simulink model "main_adaptive"  (R2021b)
settings: Solver=ode45  StartTime=0.0  StopTime=80  FixedStep=0.1  RelTol=1e-4
libraries: slpidlib x6
(part 1 of 2)
settings Model: Creator=rooz1200  LastModifiedBy=rooz1200
settings SolverCC: AlgebraicLoopSolver=TrustRegion
settings OptimizationCC: DefaultParameterBehavior=Inlined  EnhancedBackFolding=on  PassReuseOutputArgsAs=Individual arguments  ZeroExternalMemoryAtStartup=off  ZeroInternalMemoryAtStartup=off  OptimizeBlockOrder=speed  DifferentSizesBufferReuse=on  OptimizationCustomize=off  EfficientTunableParamExpr=on
settings DebuggingCC: ParameterTunabilityLossMsg=error  UnderSpecifiedDimensionMsg=warning  ArithmeticOperatorsInVariantConditions=warning
settings SFSimCC: MATLABDynamicMemAlloc=off  CustomCodeUndefinedFunction=UseInterfaceOnly
settings RTWCC: Description=Embedded Coder  SystemTargetFile=ert.tlc  GenCodeOnly=on  TemplateMakefile=ert_default_tmf
settings CodeAppCC: ForceParamTrailComments=on  IgnoreCustomStorageClasses=off  OperatorAnnotations=on  SimulinkDataObjDesc=on  SFDataObjDesc=on  InsertBlockDesc=on
settings ERTTargetCC: TargetLangStandard=C99 (ISO)  GenerateSampleERTMain=on  InlinedParameterPlacement=NonHierarchical  ERTCustomFileTemplate=example_file_process.tlc

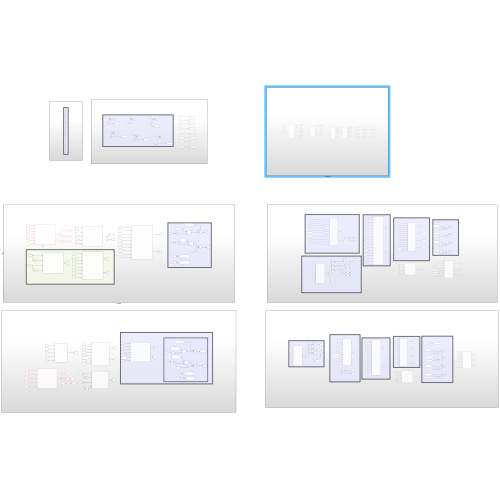
[thumbnail: Simulink's stored preview of the top-level diagram]
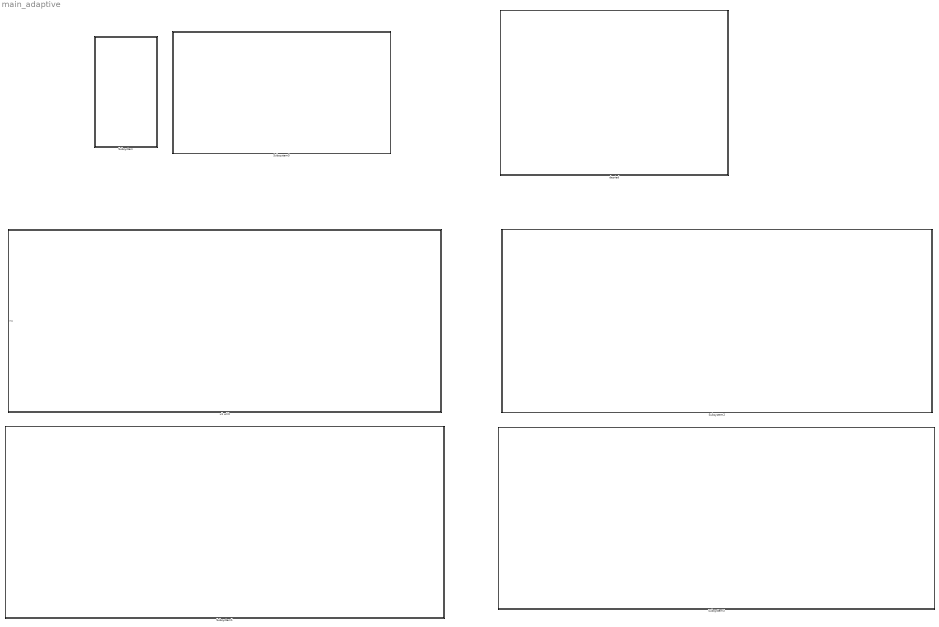
== system main_adaptive ==
  Subsystem : Subsystem
  Subsystem1 : Subsystem
  Subsystem2 : Subsystem
  Subsystem3 : Subsystem
  Subsystem5 : Subsystem
  desried : Subsystem
  "u1 whit " : Subsystem

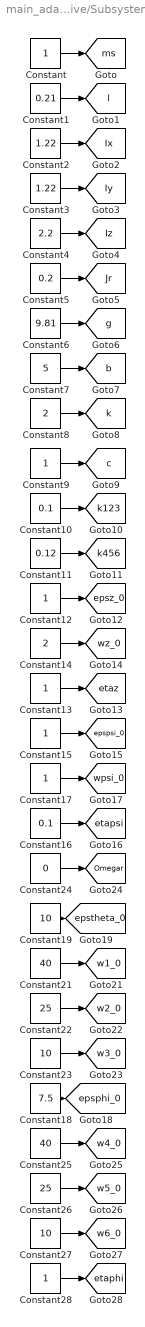
== system main_adaptive/Subsystem ==
  Constant{,9,12..13,15,17,28} (7 alike) : Constant
  Constant1 : Constant  Value=0.21
  Constant10 : Constant  Value=0.1
  Constant11 : Constant  Value=0.12
  Constant14 : Constant  Value=2
  Constant16 : Constant  Value=0.1
  Constant18 : Constant  Value=7.5
  Constant19 : Constant  Value=10
  Constant2 : Constant  Value=1.22
  Constant21 : Constant  Value=40
  Constant22 : Constant  Value=25
  Constant23 : Constant  Value=10
  Constant24 : Constant  Value=0
  Constant25 : Constant  Value=40
  Constant26 : Constant  Value=25
  Constant27 : Constant  Value=10
  Constant3 : Constant  Value=1.22
  Constant4 : Constant  Value=2.2
  Constant5 : Constant  Value=0.2
  Constant6 : Constant  Value=9.81
  Constant7 : Constant  Value=5
  Constant8 : Constant  Value=2
  tag scope: Ix=global, Iy=global, Iz=global, Jr=global, Omegar=global, b=global, c=global, epsphi_0=global, epspsi_0=global, epstheta_0=global, epsz_0=global, etaphi=global, etapsi=global, etaz=global, g=global, k123=global, k456=global, k=global, l=global, ms=global, w1_0=global, w2_0=global, w3_0=global, w4_0=global, w5_0=global, w6_0=global, wpsi_0=global, wz_0=global
  wires:
  Constant15/1 -> [epspsi_0]
  Constant4/1 -> [Iz]
  Constant11/1 -> [k456]
  Constant/1 -> [ms]
  Constant10/1 -> [k123]
  Constant22/1 -> [w2_0]
  Constant1/1 -> [l]
  Constant6/1 -> [g]
  Constant17/1 -> [wpsi_0]
  Constant13/1 -> [etaz]
  Constant21/1 -> [w1_0]
  Constant8/1 -> [k]
  Constant25/1 -> [w4_0]
  Constant23/1 -> [w3_0]
  Constant18/1 -> [epsphi_0]
  Constant3/1 -> [Iy]
  Constant2/1 -> [Ix]
  Constant16/1 -> [etapsi]
  Constant24/1 -> [Omegar]
  Constant26/1 -> [w5_0]
  Constant5/1 -> [Jr]
  Constant7/1 -> [b]
  Constant19/1 -> [epstheta_0]
  Constant14/1 -> [wz_0]
  Constant27/1 -> [w6_0]
  Constant12/1 -> [epsz_0]
  Constant9/1 -> [c]
  Constant28/1 -> [etaphi]

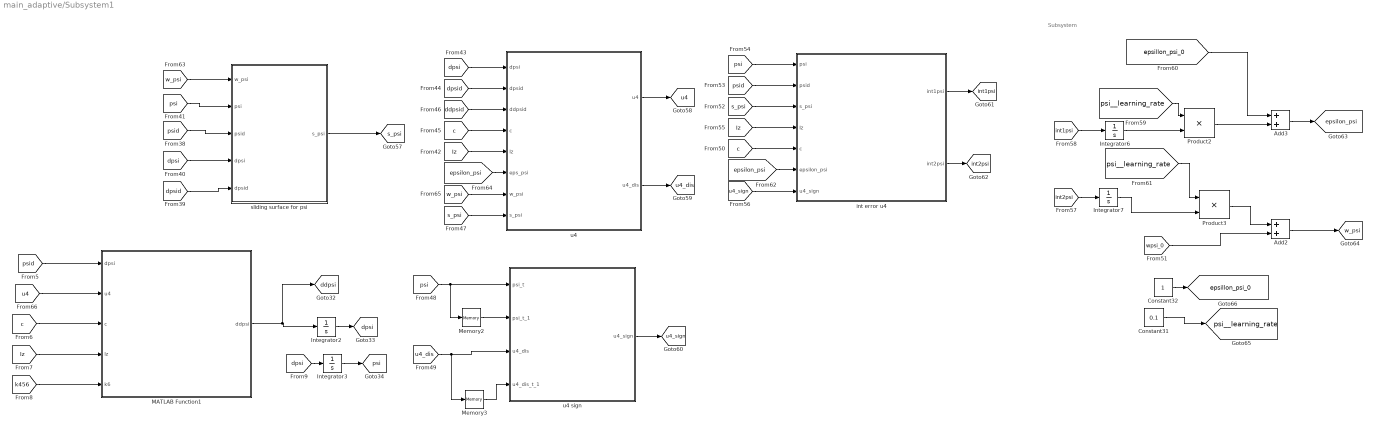
== system main_adaptive/Subsystem1 ==
  note: Subsystem
  Add2 : Sum
  Add3 : Sum
  Constant31 : Constant  Value=0.1
  Constant32 : Constant
  Integrator{2..3,6..7} (4 alike) : Integrator
  MATLAB Function1 : MATLAB Function  TreatAsAtomicUnit=on
  Memory2 : Memory
  Memory3 : Memory
  Product2 : Product
  Product3 : Product
  int error u4 : MATLAB Function  TreatAsAtomicUnit=on
  sliding surface for psi : MATLAB Function  TreatAsAtomicUnit=on
  u4 : MATLAB Function  TreatAsAtomicUnit=on
  "u4 sign " : MATLAB Function  TreatAsAtomicUnit=on
  tag scope: ddpsi=global, dpsi=global, epsillon_psi_0=global, epsilon_psi=global, int1psi=global, int2psi=global, psi=global, psi__learning_rate=global, s_psi=global, u4=global, u4_dis=global, u4_sign=global, w_psi=global
  wires:
  [psid] -> int error u4/2(psid)
  [dpsi] -> u4/1(dpsi)
  [c] -> int error u4/5(c)
  [u4_dis] -> "u4 sign "/3(u4_dis), Memory3/1
  "u4 sign "/1(u4_sign) -> [u4_sign]
  [psi] -> sliding surface for psi/2(psi)
  [w_psi] -> u4/7(w_psi)
  [dpsid] -> sliding surface for psi/5(dpsid)
  [u4_sign] -> int error u4/7(u4_sign)
  [epsilon_psi] -> int error u4/6(epsilon_psi)
  [epsilon_psi] -> u4/6(eps_psi)
  Memory3/1 -> "u4 sign "/4(u4_dis_t_1)
  sliding surface for psi/1(s_psi) -> [s_psi]
  [c] -> u4/4(c)
  [dpsi] -> sliding surface for psi/4(dpsi)
  [s_psi] -> u4/8(s_psi)
  [psi] -> int error u4/1(psi)
  u4/1(u4) -> [u4]
  [s_psi] -> int error u4/3(s_psi)
  Memory2/1 -> "u4 sign "/2(psi_t_1)
  [psi] -> "u4 sign "/1(psi_t), Memory2/1
  int error u4/1(int1psi) -> [int1psi]
  int error u4/2(int2psi) -> [int2psi]
  [ddpsid] -> u4/3(ddpsid)
  [Iz] -> int error u4/4(Iz)
  [w_psi] -> sliding surface for psi/1(w_psi)
  u4/2(u4_dis) -> [u4_dis]
  [psid] -> sliding surface for psi/3(psid)
  [dpsid] -> u4/2(dpsid)
  [Iz] -> u4/5(Iz)
  Constant32/1 -> [epsillon_psi_0]
  [psi__learning_rate] -> Product2/1
  Integrator6/1 -> Product2/2
  Product3/1 -> Add2/1
  [int1psi] -> Integrator6/1
  Add2/1 -> [w_psi]
  [wpsi_0] -> Add2/2
  Add3/1 -> [epsilon_psi]
  Integrator7/1 -> Product3/2
  [psi__learning_rate] -> Product3/1
  [int2psi] -> Integrator7/1
  Constant31/1 -> [psi__learning_rate]
  Product2/1 -> Add3/2
  [epsillon_psi_0] -> Add3/1
  [k456] -> MATLAB Function1/5(k6)
  [Iz] -> MATLAB Function1/4(Iz)
  [c] -> MATLAB Function1/3(c)
  Integrator3/1 -> [psi]
  [psid] -> MATLAB Function1/1(dpsi)
  [u4] -> MATLAB Function1/2(u4)
  MATLAB Function1/1(ddpsi) -> [ddpsi], Integrator2/1
  Integrator2/1 -> [dpsi]
  [dpsi] -> Integrator3/1

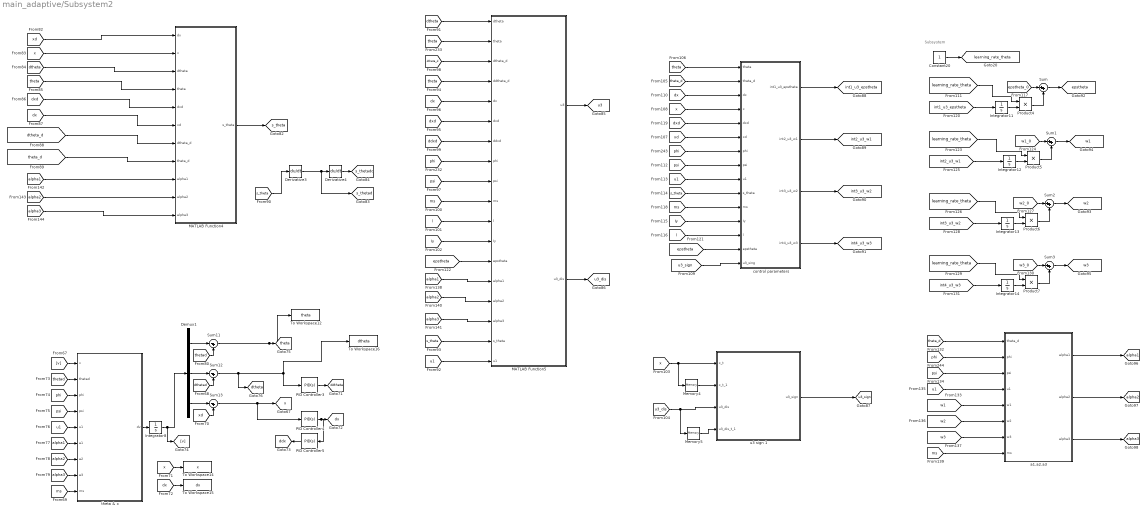
== system main_adaptive/Subsystem2 ==
  note: Subsystem
  Constant20 : Constant
  Demux1 : Demux  Outputs=3
  Derivative3 : Derivative
  Derivative4 : Derivative
  Integrator{11..14} (4 alike) : Integrator
  Integrator8 : Integrator  InitialCondition=[0;0;0.6]
  MATLAB Function4 : MATLAB Function  TreatAsAtomicUnit=on
  MATLAB Function5 : MATLAB Function  TreatAsAtomicUnit=on
  Memory4 : Memory
  Memory5 : Memory
  PID Controller3 : slpidlib/PID Controller  Controller=PID  Form=Parallel  TimeDomain=Continuous-time  UseExternalTs=off  SampleTime=-1  IntegratorMethod=Forward Euler  FilterMethod=Forward Euler  ControllerParametersSource=internal  P=0  I=0  D=1  UseFilter=on  N=100  TunerSelectOption=Transfer Function Based (PID Tuner App)  InitialConditionSource=internal  InitialConditionForIntegrator=0  InitialConditionForFilter=0  DifferentiatorICPrevScaledInput=0  ExternalReset=none  TrackingMode=off  Kt=1  LimitOutput=off  SatLimitsSource=internal  UpperSaturationLimit=inf  LowerSaturationLimit=-inf  LinearizeAsGain=on  AntiWindupMode=none  Kb=1  POutMin=[]  POutMax=[]  IOutMin=[]  IOutMax=[]  DOutMin=[]  DOutMax=[]  NOutMin=[]  NOutMax=[]  SumOutMin=[]  SumOutMax=[]  SaturationOutMin=[]  SaturationOutMax=[]  PParamMin=[]  PParamMax=[]  IParamMin=[]  IParamMax=[]  DParamMin=[]  DParamMax=[]  NParamMin=[]  NParamMax=[]  KbParamMin=[]  KbParamMax=[]  KtParamMin=[]  KtParamMax=[]  KbOutMin=[]  KbOutMax=[]  KtOutMin=[]  KtOutMax=[]  IntegratorOutMin=[]  IntegratorOutMax=[]  FilterOutMin=[]  FilterOutMax=[]  SumI1OutMin=[]  SumI1OutMax=[]  SumI2OutMin=[]  SumI2OutMax=[]  SumI3OutMin=[]  SumI3OutMax=[]  SumI4OutMin=[]  SumI4OutMax=[]  SumDOutMin=[]  SumDOutMax=[]  DifferentiatorOutMin=[]  DifferentiatorOutMax=[]  FilterDiffOutCoefMin=[]  FilterDiffOutCoefMax=[]  ReciprocalOutMin=[]  ReciprocalOutMax=[]  SumDenOutMin=[]  SumDenOutMax=[]  SumNumOutMin=[]  SumNumOutMax=[]  DivideOutMin=[]  DivideOutMax=[]  UdiffTsProdOutMin=[]  UdiffTsProdOutMax=[]  NTsProdOutMin=[]  NTsProdOutMax=[]  UintegralTsProdOutMin=[]  UintegralTsProdOutMax=[]  UngainTsProdOutMin=[]  UngainTsProdOutMax=[]  IntegratorContinuousStateAttributes=''  IntegratorStateMustResolveToSignalObject=off  IntegratorRTWStateStorageClass=Auto  FilterContinuousStateAttributes=''  FilterStateMustResolveToSignalObject=off  FilterRTWStateStorageClass=Auto  ParallelPVariant=InternalParameters  IdealPVariant=Disabled  IVariant=InternalParameters  DVariant=InternalParameters  IntegratorVariant=Continuous  SatVariant=Disabled  AWVariant=Passthrough  PCopyVariant=Disabled  TRVariant=Disabled  FdbkBlocksVariant=Forward  IdealPFdbkVariant=Disabled  SatFdbkVariant=Disabled  DerivativeFilterVariant=ContFilter  NVariant=InternalParameters  NCopyVariant=Disabled  FilterICVariant=InternalICsFilter  IntegratorICVariant=InternalICs  ExternalResetVariant=Disabled  TRSumVariant=Passthrough  SumFdbkVariant=Disabled  SumVariant=Sum_PID  TsampFilterVariant=InternalTs  TsampNgainVariant=Passthrough  TsampIntegralVariant=Passthrough  ExternalSaturationOutDataTypeStr=Inherit: Same as second input
  PID Controller4 : slpidlib/PID Controller  Controller=PID  Form=Parallel  TimeDomain=Continuous-time  UseExternalTs=off  SampleTime=-1  IntegratorMethod=Forward Euler  FilterMethod=Forward Euler  ControllerParametersSource=internal  P=0  I=0  D=1  UseFilter=on  N=100  TunerSelectOption=Transfer Function Based (PID Tuner App)  InitialConditionSource=internal  InitialConditionForIntegrator=0  InitialConditionForFilter=0  DifferentiatorICPrevScaledInput=0  ExternalReset=none  TrackingMode=off  Kt=1  LimitOutput=off  SatLimitsSource=internal  UpperSaturationLimit=inf  LowerSaturationLimit=-inf  LinearizeAsGain=on  AntiWindupMode=none  Kb=1  POutMin=[]  POutMax=[]  IOutMin=[]  IOutMax=[]  DOutMin=[]  DOutMax=[]  NOutMin=[]  NOutMax=[]  SumOutMin=[]  SumOutMax=[]  SaturationOutMin=[]  SaturationOutMax=[]  PParamMin=[]  PParamMax=[]  IParamMin=[]  IParamMax=[]  DParamMin=[]  DParamMax=[]  NParamMin=[]  NParamMax=[]  KbParamMin=[]  KbParamMax=[]  KtParamMin=[]  KtParamMax=[]  KbOutMin=[]  KbOutMax=[]  KtOutMin=[]  KtOutMax=[]  IntegratorOutMin=[]  IntegratorOutMax=[]  FilterOutMin=[]  FilterOutMax=[]  SumI1OutMin=[]  SumI1OutMax=[]  SumI2OutMin=[]  SumI2OutMax=[]  SumI3OutMin=[]  SumI3OutMax=[]  SumI4OutMin=[]  SumI4OutMax=[]  SumDOutMin=[]  SumDOutMax=[]  DifferentiatorOutMin=[]  DifferentiatorOutMax=[]  FilterDiffOutCoefMin=[]  FilterDiffOutCoefMax=[]  ReciprocalOutMin=[]  ReciprocalOutMax=[]  SumDenOutMin=[]  SumDenOutMax=[]  SumNumOutMin=[]  SumNumOutMax=[]  DivideOutMin=[]  DivideOutMax=[]  UdiffTsProdOutMin=[]  UdiffTsProdOutMax=[]  NTsProdOutMin=[]  NTsProdOutMax=[]  UintegralTsProdOutMin=[]  UintegralTsProdOutMax=[]  UngainTsProdOutMin=[]  UngainTsProdOutMax=[]  IntegratorContinuousStateAttributes=''  IntegratorStateMustResolveToSignalObject=off  IntegratorRTWStateStorageClass=Auto  FilterContinuousStateAttributes=''  FilterStateMustResolveToSignalObject=off  FilterRTWStateStorageClass=Auto  ParallelPVariant=InternalParameters  IdealPVariant=Disabled  IVariant=InternalParameters  DVariant=InternalParameters  IntegratorVariant=Continuous  SatVariant=Disabled  AWVariant=Passthrough  PCopyVariant=Disabled  TRVariant=Disabled  FdbkBlocksVariant=Forward  IdealPFdbkVariant=Disabled  SatFdbkVariant=Disabled  DerivativeFilterVariant=ContFilter  NVariant=InternalParameters  NCopyVariant=Disabled  FilterICVariant=InternalICsFilter  IntegratorICVariant=InternalICs  ExternalResetVariant=Disabled  TRSumVariant=Passthrough  SumFdbkVariant=Disabled  SumVariant=Sum_PID  TsampFilterVariant=InternalTs  TsampNgainVariant=Passthrough  TsampIntegralVariant=Passthrough  ExternalSaturationOutDataTypeStr=Inherit: Same as second input
  PID Controller5 : slpidlib/PID Controller  Controller=PID  Form=Parallel  TimeDomain=Continuous-time  UseExternalTs=off  SampleTime=-1  IntegratorMethod=Forward Euler  FilterMethod=Forward Euler  ControllerParametersSource=internal  P=0  I=0  D=1  UseFilter=on  N=100  TunerSelectOption=Transfer Function Based (PID Tuner App)  InitialConditionSource=internal  InitialConditionForIntegrator=0  InitialConditionForFilter=0  DifferentiatorICPrevScaledInput=0  ExternalReset=none  TrackingMode=off  Kt=1  LimitOutput=off  SatLimitsSource=internal  UpperSaturationLimit=inf  LowerSaturationLimit=-inf  LinearizeAsGain=on  AntiWindupMode=none  Kb=1  POutMin=[]  POutMax=[]  IOutMin=[]  IOutMax=[]  DOutMin=[]  DOutMax=[]  NOutMin=[]  NOutMax=[]  SumOutMin=[]  SumOutMax=[]  SaturationOutMin=[]  SaturationOutMax=[]  PParamMin=[]  PParamMax=[]  IParamMin=[]  IParamMax=[]  DParamMin=[]  DParamMax=[]  NParamMin=[]  NParamMax=[]  KbParamMin=[]  KbParamMax=[]  KtParamMin=[]  KtParamMax=[]  KbOutMin=[]  KbOutMax=[]  KtOutMin=[]  KtOutMax=[]  IntegratorOutMin=[]  IntegratorOutMax=[]  FilterOutMin=[]  FilterOutMax=[]  SumI1OutMin=[]  SumI1OutMax=[]  SumI2OutMin=[]  SumI2OutMax=[]  SumI3OutMin=[]  SumI3OutMax=[]  SumI4OutMin=[]  SumI4OutMax=[]  SumDOutMin=[]  SumDOutMax=[]  DifferentiatorOutMin=[]  DifferentiatorOutMax=[]  FilterDiffOutCoefMin=[]  FilterDiffOutCoefMax=[]  ReciprocalOutMin=[]  ReciprocalOutMax=[]  SumDenOutMin=[]  SumDenOutMax=[]  SumNumOutMin=[]  SumNumOutMax=[]  DivideOutMin=[]  DivideOutMax=[]  UdiffTsProdOutMin=[]  UdiffTsProdOutMax=[]  NTsProdOutMin=[]  NTsProdOutMax=[]  UintegralTsProdOutMin=[]  UintegralTsProdOutMax=[]  UngainTsProdOutMin=[]  UngainTsProdOutMax=[]  IntegratorContinuousStateAttributes=''  IntegratorStateMustResolveToSignalObject=off  IntegratorRTWStateStorageClass=Auto  FilterContinuousStateAttributes=''  FilterStateMustResolveToSignalObject=off  FilterRTWStateStorageClass=Auto  ParallelPVariant=InternalParameters  IdealPVariant=Disabled  IVariant=InternalParameters  DVariant=InternalParameters  IntegratorVariant=Continuous  SatVariant=Disabled  AWVariant=Passthrough  PCopyVariant=Disabled  TRVariant=Disabled  FdbkBlocksVariant=Forward  IdealPFdbkVariant=Disabled  SatFdbkVariant=Disabled  DerivativeFilterVariant=ContFilter  NVariant=InternalParameters  NCopyVariant=Disabled  FilterICVariant=InternalICsFilter  IntegratorICVariant=InternalICs  ExternalResetVariant=Disabled  TRSumVariant=Passthrough  SumFdbkVariant=Disabled  SumVariant=Sum_PID  TsampFilterVariant=InternalTs  TsampNgainVariant=Passthrough  TsampIntegralVariant=Passthrough  ExternalSaturationOutDataTypeStr=Inherit: Same as second input
  Product{4..7} (4 alike) : Product
  Sum{,1..3} (4 alike) : Sum  Inputs=|++
  Sum11 : Sum  Inputs=|-+
  Sum12 : Sum  Inputs=|-+
  Sum13 : Sum  Inputs=|-+
  To Workspace12 : ToWorkspace  VariableName=theta  SampleTime=-1
      settings: Save2DSignal=2-D array (concatenate along first dimension)
  To Workspace14 : ToWorkspace  VariableName=x  SampleTime=-1
      settings: Save2DSignal=2-D array (concatenate along first dimension)
  To Workspace15 : ToWorkspace  VariableName=dx  SampleTime=-1
      settings: Save2DSignal=2-D array (concatenate along first dimension)
  To Workspace16 : ToWorkspace  VariableName=dtheta  SampleTime=-1
      settings: Save2DSignal=2-D array (concatenate along first dimension)
  a1,a2,a3 : MATLAB Function  TreatAsAtomicUnit=on
  control parameters : MATLAB Function  TreatAsAtomicUnit=on
  theta & x : MATLAB Function  TreatAsAtomicUnit=on
  u3 sign 1 : MATLAB Function  TreatAsAtomicUnit=on
  tag scope: alpha1=global, alpha2=global, alpha3=global, ddtheta=global, ddx=global, dtheta=global, dx=global, epstheta=global, int1_u3_epstheta=global, int2_u3_w1=global, int3_u3_w2=global, int4_u3_w3=global, learning_rate_theta=global, s_theta=global, s_thetad=global, s_thetadd=global, theta=global, u3=global, u3_dis=global, u3_sign=global, w1=global, w2=global, w3=global, x=global
  wires:
  [dxd] -> MATLAB Function4/5(dxd)
  [alpha1] -> MATLAB Function4/9(alpha1)
  Memory4/1 -> u3 sign 1/2(x_t_1)
  [s_theta] -> MATLAB Function5/17(s_theta)
  Sum12/1 -> To Workspace16/1, PID Controller3/1, [dtheta]
  [theta] -> MATLAB Function5/2(theta)
  [phi] -> a1,a2,a3/2(phi)
  control parameters/4(int4_u3_w3) -> [int4_u3_w3]
  PID Controller5/1 -> [ddx]
  MATLAB Function5/1(u3) -> [u3]
  [ms] -> control parameters/11(ms)
  [theta] -> MATLAB Function5/4(ddtheta_d)
  [w2] -> a1,a2,a3/6(w2)
  Derivative4/1 -> [s_thetadd]
  [epstheta] -> control parameters/14(epstheta)
  [u3_sign] -> control parameters/15(u3_sing)
  [theta_d] -> control parameters/2(theta_d)
  [ms] -> MATLAB Function5/10(ms)
  [ddxd] -> MATLAB Function5/7(ddxd)
  Demux1/2 -> Sum12/1
  Sum11/1 -> To Workspace12/1, [theta]
  [theta_d] -> a1,a2,a3/1(theta_d)
  [alpha2] -> MATLAB Function4/10(alpha2)
  [thetad] -> Sum11/2
  [dxd] -> MATLAB Function5/6(dxd)
  [thetad] -> theta & x/2(thetad)
  a1,a2,a3/2(alpha2) -> [alpha2]
  [alpha1] -> MATLAB Function5/14(alpha1)
  [psi] -> theta & x/4(psi)
  [dtheta] -> MATLAB Function4/3(dtheta)
  Memory5/1 -> u3 sign 1/4(u3_dis_t_1)
  [ms] -> theta & x/9(ms)
  theta & x/1(dv) -> Integrator8/1
  [xd] -> control parameters/6(xd)
  Sum13/1 -> [x], PID Controller4/1
  [s_theta] -> Derivative3/1
  [alpha1] -> theta & x/6(a1)
  [phi] -> theta & x/3(phi)
  [dx] -> MATLAB Function5/5(dx)
  [psi] -> MATLAB Function5/9(psi)
  control parameters/3(int3_u3_w2) -> [int3_u3_w2]
  [alpha3] -> MATLAB Function4/11(alpha3)
  [x] -> u3 sign 1/1(x_t), Memory4/1
  [alpha2] -> MATLAB Function5/15(alpha2)
  [Iy] -> MATLAB Function5/12(Iy)
  [l] -> control parameters/13(l)
  [psi] -> control parameters/8(psi)
  [dtheta] -> MATLAB Function5/1(dtheta)
  MATLAB Function5/2(u3_dis) -> [u3_dis]
  MATLAB Function4/1(s_theta) -> [s_theta]
  [dtheta_d] -> MATLAB Function4/7(dtheta_d)
  [Iy] -> control parameters/12(Iy)
  [x] -> control parameters/4(x)
  [u1] -> control parameters/9(u1)
  [dtheta_d] -> MATLAB Function5/3(dtheta_d)
  [u1] -> MATLAB Function5/18(u1)
  [dx] -> MATLAB Function4/6(xd)
  control parameters/1(int1_u3_epstheta) -> [int1_u3_epstheta]
  [theta] -> MATLAB Function4/4(theta)
  [phi] -> MATLAB Function5/8(phi)
  [dthetad] -> Sum12/2
  [ms] -> a1,a2,a3/8(ms)
  control parameters/2(int2_u3_w1) -> [int2_u3_w1]
  [u3_dis] -> u3 sign 1/3(u3_dis), Memory5/1
  Derivative3/1 -> Derivative4/1, [s_thetad]
  a1,a2,a3/3(alpha3) -> [alpha3]
  [theta] -> control parameters/1(theta)
  [w3] -> a1,a2,a3/7(w3)
  a1,a2,a3/1(alpha1) -> [alpha1]
  [dx] -> control parameters/3(dx)
  [psi] -> a1,a2,a3/3(psi)
  [theta_d] -> MATLAB Function4/8(theta_d)
  [alpha3] -> MATLAB Function5/16(alpha3)
  u3 sign 1/1(u3_sign) -> [u3_sign]
  [phi] -> control parameters/7(phi)
  [w1] -> a1,a2,a3/5(w1)
  [u1] -> a1,a2,a3/4(u1)
  Demux1/3 -> Sum13/1
  [v] -> theta & x/1(v)
  PID Controller4/1 -> PID Controller5/1, [dx]
  [s_theta] -> control parameters/10(s_theta)
  [x] -> To Workspace14/1
  [dx] -> To Workspace15/1
  Integrator8/1 -> Demux1/1, [v]
  PID Controller3/1 -> [ddtheta]
  [alpha3] -> theta & x/8(a3)
  [x] -> MATLAB Function4/2(x)
  [u1] -> theta & x/5(u1)
  [alpha2] -> theta & x/7(a2)
  Demux1/1 -> Sum11/1
  [xd] -> Sum13/2
  [dxd] -> control parameters/5(dxd)
  [xd] -> MATLAB Function4/1(dx)
  [epstheta] -> MATLAB Function5/13(epstheta)
  [l] -> MATLAB Function5/11(l)
  [learning_rate_theta] -> Product7/1
  [w1_0] -> Sum1/1
  Sum1/1 -> [w1]
  Product6/1 -> Sum2/2
  Sum/1 -> [epstheta]
  Product4/1 -> Sum/2
  Sum2/1 -> [w2]
  Product5/1 -> Sum1/2
  [learning_rate_theta] -> Product4/1
  Constant20/1 -> [learning_rate_theta]
  [int2_u3_w1] -> Integrator12/1
  Integrator13/1 -> Product6/2
  Product7/1 -> Sum3/2
  Integrator14/1 -> Product7/2
  Sum3/1 -> [w3]
  [int3_u3_w2] -> Integrator13/1
  [int4_u3_w3] -> Integrator14/1
  [w3_0] -> Sum3/1
  Integrator12/1 -> Product5/2
  [epstheta_0] -> Sum/1
  [w2_0] -> Sum2/1
  [int1_u3_epstheta] -> Integrator11/1
  [learning_rate_theta] -> Product6/1
  Integrator11/1 -> Product4/2
  [learning_rate_theta] -> Product5/1

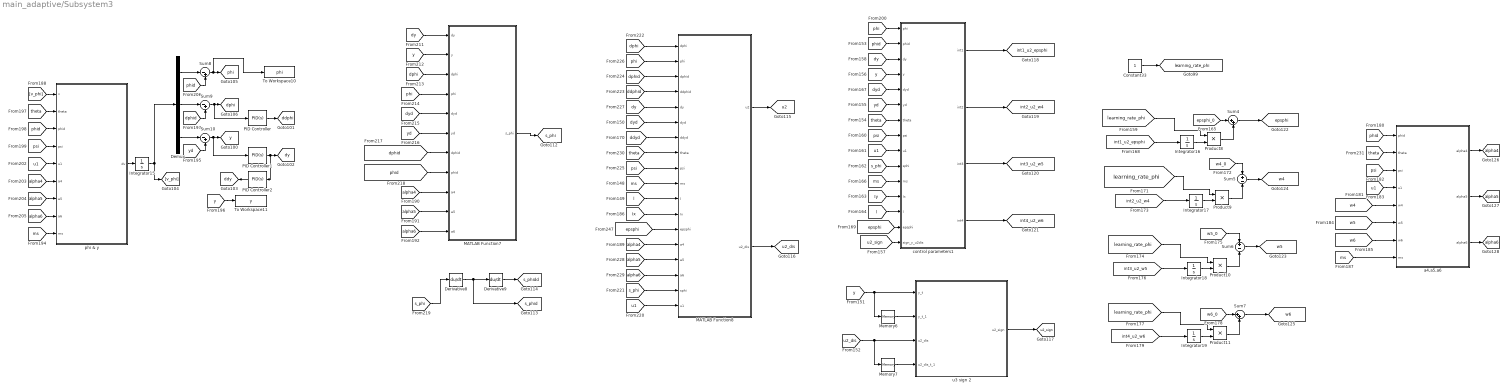
== system main_adaptive/Subsystem3 ==
  Constant33 : Constant
  Demux : Demux  Outputs=3
  Derivative8 : Derivative
  Derivative9 : Derivative
  Integrator15 : Integrator  InitialCondition=[0;0;0.6]
  Integrator{16..19} (4 alike) : Integrator
  MATLAB Function7 : MATLAB Function  TreatAsAtomicUnit=on
  MATLAB Function8 : MATLAB Function  TreatAsAtomicUnit=on
  Memory6 : Memory
  Memory7 : Memory
  PID Controller : slpidlib/PID Controller  Controller=PID  Form=Parallel  TimeDomain=Continuous-time  UseExternalTs=off  SampleTime=-1  IntegratorMethod=Forward Euler  FilterMethod=Forward Euler  ControllerParametersSource=internal  P=0  I=0  D=1  UseFilter=on  N=100  TunerSelectOption=Transfer Function Based (PID Tuner App)  InitialConditionSource=internal  InitialConditionForIntegrator=0  InitialConditionForFilter=0  DifferentiatorICPrevScaledInput=0  ExternalReset=none  TrackingMode=off  Kt=1  LimitOutput=off  SatLimitsSource=internal  UpperSaturationLimit=inf  LowerSaturationLimit=-inf  LinearizeAsGain=on  AntiWindupMode=none  Kb=1  POutMin=[]  POutMax=[]  IOutMin=[]  IOutMax=[]  DOutMin=[]  DOutMax=[]  NOutMin=[]  NOutMax=[]  SumOutMin=[]  SumOutMax=[]  SaturationOutMin=[]  SaturationOutMax=[]  PParamMin=[]  PParamMax=[]  IParamMin=[]  IParamMax=[]  DParamMin=[]  DParamMax=[]  NParamMin=[]  NParamMax=[]  KbParamMin=[]  KbParamMax=[]  KtParamMin=[]  KtParamMax=[]  KbOutMin=[]  KbOutMax=[]  KtOutMin=[]  KtOutMax=[]  IntegratorOutMin=[]  IntegratorOutMax=[]  FilterOutMin=[]  FilterOutMax=[]  SumI1OutMin=[]  SumI1OutMax=[]  SumI2OutMin=[]  SumI2OutMax=[]  SumI3OutMin=[]  SumI3OutMax=[]  SumI4OutMin=[]  SumI4OutMax=[]  SumDOutMin=[]  SumDOutMax=[]  DifferentiatorOutMin=[]  DifferentiatorOutMax=[]  FilterDiffOutCoefMin=[]  FilterDiffOutCoefMax=[]  ReciprocalOutMin=[]  ReciprocalOutMax=[]  SumDenOutMin=[]  SumDenOutMax=[]  SumNumOutMin=[]  SumNumOutMax=[]  DivideOutMin=[]  DivideOutMax=[]  UdiffTsProdOutMin=[]  UdiffTsProdOutMax=[]  NTsProdOutMin=[]  NTsProdOutMax=[]  UintegralTsProdOutMin=[]  UintegralTsProdOutMax=[]  UngainTsProdOutMin=[]  UngainTsProdOutMax=[]  IntegratorContinuousStateAttributes=''  IntegratorStateMustResolveToSignalObject=off  IntegratorRTWStateStorageClass=Auto  FilterContinuousStateAttributes=''  FilterStateMustResolveToSignalObject=off  FilterRTWStateStorageClass=Auto  ParallelPVariant=InternalParameters  IdealPVariant=Disabled  IVariant=InternalParameters  DVariant=InternalParameters  IntegratorVariant=Continuous  SatVariant=Disabled  AWVariant=Passthrough  PCopyVariant=Disabled  TRVariant=Disabled  FdbkBlocksVariant=Forward  IdealPFdbkVariant=Disabled  SatFdbkVariant=Disabled  DerivativeFilterVariant=ContFilter  NVariant=InternalParameters  NCopyVariant=Disabled  FilterICVariant=InternalICsFilter  IntegratorICVariant=InternalICs  ExternalResetVariant=Disabled  TRSumVariant=Passthrough  SumFdbkVariant=Disabled  SumVariant=Sum_PID  TsampFilterVariant=InternalTs  TsampNgainVariant=Passthrough  TsampIntegralVariant=Passthrough  ExternalSaturationOutDataTypeStr=Inherit: Same as second input
  PID Controller1 : slpidlib/PID Controller  Controller=PID  Form=Parallel  TimeDomain=Continuous-time  UseExternalTs=off  SampleTime=-1  IntegratorMethod=Forward Euler  FilterMethod=Forward Euler  ControllerParametersSource=internal  P=0  I=0  D=1  UseFilter=on  N=100  TunerSelectOption=Transfer Function Based (PID Tuner App)  InitialConditionSource=internal  InitialConditionForIntegrator=0  InitialConditionForFilter=0  DifferentiatorICPrevScaledInput=0  ExternalReset=none  TrackingMode=off  Kt=1  LimitOutput=off  SatLimitsSource=internal  UpperSaturationLimit=inf  LowerSaturationLimit=-inf  LinearizeAsGain=on  AntiWindupMode=none  Kb=1  POutMin=[]  POutMax=[]  IOutMin=[]  IOutMax=[]  DOutMin=[]  DOutMax=[]  NOutMin=[]  NOutMax=[]  SumOutMin=[]  SumOutMax=[]  SaturationOutMin=[]  SaturationOutMax=[]  PParamMin=[]  PParamMax=[]  IParamMin=[]  IParamMax=[]  DParamMin=[]  DParamMax=[]  NParamMin=[]  NParamMax=[]  KbParamMin=[]  KbParamMax=[]  KtParamMin=[]  KtParamMax=[]  KbOutMin=[]  KbOutMax=[]  KtOutMin=[]  KtOutMax=[]  IntegratorOutMin=[]  IntegratorOutMax=[]  FilterOutMin=[]  FilterOutMax=[]  SumI1OutMin=[]  SumI1OutMax=[]  SumI2OutMin=[]  SumI2OutMax=[]  SumI3OutMin=[]  SumI3OutMax=[]  SumI4OutMin=[]  SumI4OutMax=[]  SumDOutMin=[]  SumDOutMax=[]  DifferentiatorOutMin=[]  DifferentiatorOutMax=[]  FilterDiffOutCoefMin=[]  FilterDiffOutCoefMax=[]  ReciprocalOutMin=[]  ReciprocalOutMax=[]  SumDenOutMin=[]  SumDenOutMax=[]  SumNumOutMin=[]  SumNumOutMax=[]  DivideOutMin=[]  DivideOutMax=[]  UdiffTsProdOutMin=[]  UdiffTsProdOutMax=[]  NTsProdOutMin=[]  NTsProdOutMax=[]  UintegralTsProdOutMin=[]  UintegralTsProdOutMax=[]  UngainTsProdOutMin=[]  UngainTsProdOutMax=[]  IntegratorContinuousStateAttributes=''  IntegratorStateMustResolveToSignalObject=off  IntegratorRTWStateStorageClass=Auto  FilterContinuousStateAttributes=''  FilterStateMustResolveToSignalObject=off  FilterRTWStateStorageClass=Auto  ParallelPVariant=InternalParameters  IdealPVariant=Disabled  IVariant=InternalParameters  DVariant=InternalParameters  IntegratorVariant=Continuous  SatVariant=Disabled  AWVariant=Passthrough  PCopyVariant=Disabled  TRVariant=Disabled  FdbkBlocksVariant=Forward  IdealPFdbkVariant=Disabled  SatFdbkVariant=Disabled  DerivativeFilterVariant=ContFilter  NVariant=InternalParameters  NCopyVariant=Disabled  FilterICVariant=InternalICsFilter  IntegratorICVariant=InternalICs  ExternalResetVariant=Disabled  TRSumVariant=Passthrough  SumFdbkVariant=Disabled  SumVariant=Sum_PID  TsampFilterVariant=InternalTs  TsampNgainVariant=Passthrough  TsampIntegralVariant=Passthrough  ExternalSaturationOutDataTypeStr=Inherit: Same as second input
  PID Controller2 : slpidlib/PID Controller  Controller=PID  Form=Parallel  TimeDomain=Continuous-time  UseExternalTs=off  SampleTime=-1  IntegratorMethod=Forward Euler  FilterMethod=Forward Euler  ControllerParametersSource=internal  P=0  I=0  D=1  UseFilter=on  N=100  TunerSelectOption=Transfer Function Based (PID Tuner App)  InitialConditionSource=internal  InitialConditionForIntegrator=0  InitialConditionForFilter=0  DifferentiatorICPrevScaledInput=0  ExternalReset=none  TrackingMode=off  Kt=1  LimitOutput=off  SatLimitsSource=internal  UpperSaturationLimit=inf  LowerSaturationLimit=-inf  LinearizeAsGain=on  AntiWindupMode=none  Kb=1  POutMin=[]  POutMax=[]  IOutMin=[]  IOutMax=[]  DOutMin=[]  DOutMax=[]  NOutMin=[]  NOutMax=[]  SumOutMin=[]  SumOutMax=[]  SaturationOutMin=[]  SaturationOutMax=[]  PParamMin=[]  PParamMax=[]  IParamMin=[]  IParamMax=[]  DParamMin=[]  DParamMax=[]  NParamMin=[]  NParamMax=[]  KbParamMin=[]  KbParamMax=[]  KtParamMin=[]  KtParamMax=[]  KbOutMin=[]  KbOutMax=[]  KtOutMin=[]  KtOutMax=[]  IntegratorOutMin=[]  IntegratorOutMax=[]  FilterOutMin=[]  FilterOutMax=[]  SumI1OutMin=[]  SumI1OutMax=[]  SumI2OutMin=[]  SumI2OutMax=[]  SumI3OutMin=[]  SumI3OutMax=[]  SumI4OutMin=[]  SumI4OutMax=[]  SumDOutMin=[]  SumDOutMax=[]  DifferentiatorOutMin=[]  DifferentiatorOutMax=[]  FilterDiffOutCoefMin=[]  FilterDiffOutCoefMax=[]  ReciprocalOutMin=[]  ReciprocalOutMax=[]  SumDenOutMin=[]  SumDenOutMax=[]  SumNumOutMin=[]  SumNumOutMax=[]  DivideOutMin=[]  DivideOutMax=[]  UdiffTsProdOutMin=[]  UdiffTsProdOutMax=[]  NTsProdOutMin=[]  NTsProdOutMax=[]  UintegralTsProdOutMin=[]  UintegralTsProdOutMax=[]  UngainTsProdOutMin=[]  UngainTsProdOutMax=[]  IntegratorContinuousStateAttributes=''  IntegratorStateMustResolveToSignalObject=off  IntegratorRTWStateStorageClass=Auto  FilterContinuousStateAttributes=''  FilterStateMustResolveToSignalObject=off  FilterRTWStateStorageClass=Auto  ParallelPVariant=InternalParameters  IdealPVariant=Disabled  IVariant=InternalParameters  DVariant=InternalParameters  IntegratorVariant=Continuous  SatVariant=Disabled  AWVariant=Passthrough  PCopyVariant=Disabled  TRVariant=Disabled  FdbkBlocksVariant=Forward  IdealPFdbkVariant=Disabled  SatFdbkVariant=Disabled  DerivativeFilterVariant=ContFilter  NVariant=InternalParameters  NCopyVariant=Disabled  FilterICVariant=InternalICsFilter  IntegratorICVariant=InternalICs  ExternalResetVariant=Disabled  TRSumVariant=Passthrough  SumFdbkVariant=Disabled  SumVariant=Sum_PID  TsampFilterVariant=InternalTs  TsampNgainVariant=Passthrough  TsampIntegralVariant=Passthrough  ExternalSaturationOutDataTypeStr=Inherit: Same as second input
  Product{8..11} (4 alike) : Product
  Sum10 : Sum  Inputs=|-+
  Sum4 : Sum  Inputs=|++
  Sum5 : Sum  Inputs=+-
  Sum6 : Sum  Inputs=+-
  Sum7 : Sum  Inputs=|++
  Sum8 : Sum  Inputs=|-+
  Sum9 : Sum  Inputs=|-+
  To Workspace10 : ToWorkspace  VariableName=phi  SampleTime=-1
      settings: Save2DSignal=2-D array (concatenate along first dimension)
  To Workspace11 : ToWorkspace  VariableName=y  SampleTime=-1
      settings: Save2DSignal=2-D array (concatenate along first dimension)
  a4,a5,a6 : MATLAB Function  TreatAsAtomicUnit=on
  control parameters1 : MATLAB Function  TreatAsAtomicUnit=on
  phi & y : MATLAB Function  TreatAsAtomicUnit=on
  u3 sign 2 : MATLAB Function  TreatAsAtomicUnit=on
  tag scope: alpha4=global, alpha5=global, alpha6=global, ddphi=global, ddy=global, dphi=global, dy=global, epsphi=global, int1_u2_epsphi=global, int2_u2_w4=global, int3_u2_w5=global, int4_u2_w6=global, learning_rate_phi=global, phi=global, s_phi=global, s_phid=global, s_phidd=global, u2=global, u2_dis=global, u2_sign=global, w4=global, w5=global, w6=global, y=global
  wires:
  Integrator18/1 -> Product10/2
  [u2_sign] -> control parameters1/15(sign_y_u2dis)
  [int1_u2_epsphi] -> Integrator16/1
  [learning_rate_phi] -> Product9/1
  [u2_dis] -> Memory7/1, u3 sign 2/3(u2_dis)
  PID Controller2/1 -> [ddy]
  Integrator19/1 -> Product11/2
  [l] -> MATLAB Function8/11(l)
  Sum9/1 -> PID Controller/1, [dphi]
  [y] -> control parameters1/4(y)
  [y] -> u3 sign 2/1(y_t), Memory6/1
  [s_phi] -> control parameters1/10(sphi)
  [phid] -> Sum8/2
  [dphi] -> MATLAB Function7/3(dphi)
  [phi] -> MATLAB Function7/4(phi)
  [dyd] -> MATLAB Function7/5(dyd)
  [w5_0] -> Sum6/1
  [epsphi_0] -> Sum4/1
  [ms] -> phi & y/9(ms)
  Sum7/1 -> [w6]
  a4,a5,a6/1(alpha4) -> [alpha4]
  Derivative8/1 -> Derivative9/1, [s_phid]
  [alpha4] -> MATLAB Function8/14(a4)
  [alpha5] -> MATLAB Function8/15(a5)
  Memory7/1 -> u3 sign 2/4(u2_dis_t_1)
  [psi] -> MATLAB Function8/9(psi)
  [epsphi] -> control parameters1/14(epsphi)
  Constant33/1 -> [learning_rate_phi]
  [w4_0] -> Sum5/1
  control parameters1/2(int2) -> [int2_u2_w4]
  MATLAB Function7/1(s_phi) -> [s_phi]
  Sum8/1 -> To Workspace10/1, [phi]
  [alpha5] -> phi & y/7(a5)
  [phid] -> MATLAB Function7/8(phid)
  Sum10/1 -> PID Controller1/1, [y]
  [learning_rate_phi] -> Product8/1
  [Iy] -> control parameters1/12(Ix)
  Sum6/1 -> [w5]
  [alpha5] -> MATLAB Function7/10(a5)
  [ms] -> MATLAB Function8/10(ms)
  control parameters1/1(int1) -> [int1_u2_epsphi]
  [theta] -> phi & y/2(theta)
  PID Controller1/1 -> PID Controller2/1, [dy]
  [dyd] -> control parameters1/5(dyd)
  Derivative9/1 -> [s_phidd]
  [dphid] -> MATLAB Function7/7(dphid)
  [u1] -> control parameters1/9(u1)
  [learning_rate_phi] -> Product10/1
  [w6] -> a4,a5,a6/7(w6)
  [dy] -> MATLAB Function8/5(dy)
  [theta] -> MATLAB Function8/8(theta)
  [Ix] -> MATLAB Function8/12(Ix)
  Product8/1 -> Sum4/2
  [w4] -> a4,a5,a6/5(w4)
  Memory6/1 -> u3 sign 2/2(y_t_1)
  a4,a5,a6/2(alpha5) -> [alpha5]
  [ms] -> a4,a5,a6/8(ms)
  [u1] -> MATLAB Function8/18(u1)
  Integrator16/1 -> Product8/2
  [dy] -> control parameters1/3(dy)
  control parameters1/4(int4) -> [int4_u2_w6]
  [v_phi] -> phi & y/1(v)
  [w5] -> a4,a5,a6/6(w5)
  [learning_rate_phi] -> Product11/1
  [ddphid] -> MATLAB Function8/4(ddphid)
  [y] -> MATLAB Function7/2(y)
  [phi] -> control parameters1/1(phi)
  [w6_0] -> Sum7/1
  [int2_u2_w4] -> Integrator17/1
  u3 sign 2/1(u2_sign) -> [u2_sign]
  [theta] -> control parameters1/7(theta)
  [dphid] -> Sum9/2
  [psi] -> control parameters1/8(psi)
  a4,a5,a6/3(alpha6) -> [alpha6]
  PID Controller/1 -> [ddphi]
  [u1] -> a4,a5,a6/4(u1)
  Demux/2 -> Sum9/1
  [yd] -> MATLAB Function7/6(yd)
  [alpha4] -> MATLAB Function7/9(a4)
  [dyd] -> MATLAB Function8/6(dyd)
  [phid] -> control parameters1/2(phid)
  [l] -> control parameters1/13(l)
  [int4_u2_w6] -> Integrator19/1
  [ddyd] -> MATLAB Function8/7(ddyd)
  [yd] -> control parameters1/6(yd)
  Integrator15/1 -> Demux/1, [v_phi]
  MATLAB Function8/2(u2_dis) -> [u2_dis]
  [ms] -> control parameters1/11(ms)
  [psi] -> a4,a5,a6/3(psi)
  [s_phi] -> Derivative8/1
  Product11/1 -> Sum7/2
  [y] -> To Workspace11/1
  Sum4/1 -> [epsphi]
  [alpha6] -> MATLAB Function7/11(a6)
  Integrator17/1 -> Product9/2
  Demux/3 -> Sum10/1
  [alpha6] -> phi & y/8(a6)
  [psi] -> phi & y/4(psi)
  [alpha4] -> phi & y/6(a4)
  [u1] -> phi & y/5(u1)
  phi & y/1(dv) -> Integrator15/1
  [yd] -> Sum10/2
  [phid] -> a4,a5,a6/1(phid)
  [dphi] -> MATLAB Function8/1(dphi)
  [s_phi] -> MATLAB Function8/17(sphi)
  [dphid] -> MATLAB Function8/3(dphid)
  Demux/1 -> Sum8/1
  [phid] -> phi & y/3(phid)
  [epsphi] -> MATLAB Function8/13(epsphi)
  [phi] -> MATLAB Function8/2(phi)
  MATLAB Function8/1(u2) -> [u2]
  [alpha6] -> MATLAB Function8/16(a6)
  Product9/1 -> Sum5/2
  control parameters1/3(int3) -> [int3_u2_w5]
  [int3_u2_w5] -> Integrator18/1
  Product10/1 -> Sum6/2
  [theta] -> a4,a5,a6/2(theta)
  [dy] -> MATLAB Function7/1(dy)
  Sum5/1 -> [w4]

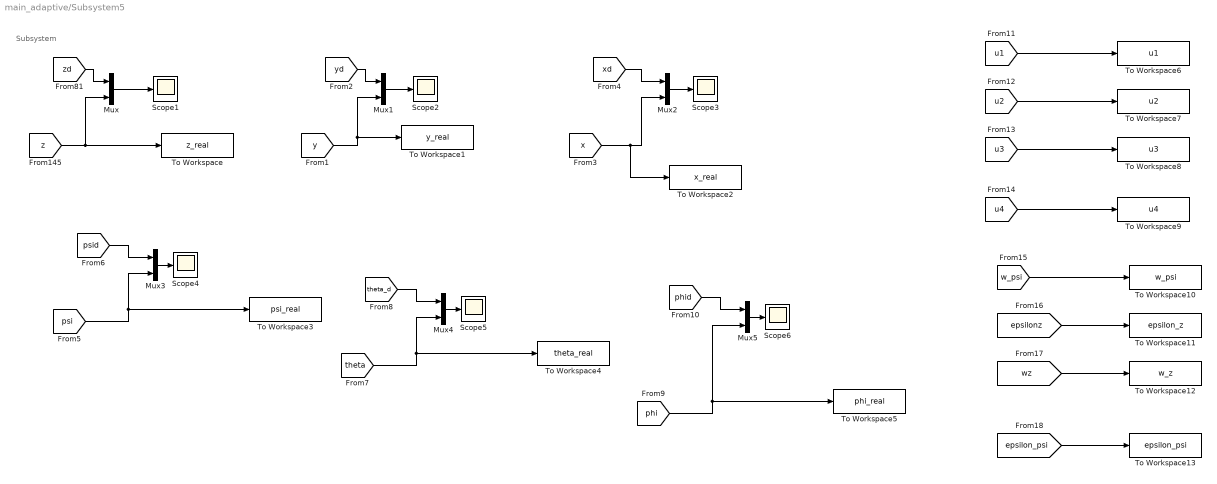
== system main_adaptive/Subsystem5 ==
  note: Subsystem
  Mux{,1..5} (6 alike) : Mux  Inputs=2
  Scope{1..6} (6 alike) : Scope
  To Workspace : ToWorkspace  VariableName=z_real  SaveFormat=Timeseries  SampleTime=-1
  To Workspace1 : ToWorkspace  VariableName=y_real  SaveFormat=Timeseries  SampleTime=-1
  To Workspace10 : ToWorkspace  VariableName=w_psi  SaveFormat=Timeseries  SampleTime=-1
  To Workspace11 : ToWorkspace  VariableName=epsilon_z  SaveFormat=Timeseries  SampleTime=-1
  To Workspace12 : ToWorkspace  VariableName=w_z  SaveFormat=Timeseries  SampleTime=-1
  To Workspace13 : ToWorkspace  VariableName=epsilon_psi  SaveFormat=Timeseries  SampleTime=-1
  To Workspace2 : ToWorkspace  VariableName=x_real  SaveFormat=Timeseries  SampleTime=-1
  To Workspace3 : ToWorkspace  VariableName=psi_real  SaveFormat=Timeseries  SampleTime=-1
  To Workspace4 : ToWorkspace  VariableName=theta_real  SaveFormat=Timeseries  SampleTime=-1
  To Workspace5 : ToWorkspace  VariableName=phi_real  SaveFormat=Timeseries  SampleTime=-1
  To Workspace6 : ToWorkspace  VariableName=u1  SaveFormat=Timeseries  SampleTime=-1
  To Workspace7 : ToWorkspace  VariableName=u2  SaveFormat=Timeseries  SampleTime=-1
  To Workspace8 : ToWorkspace  VariableName=u3  SaveFormat=Timeseries  SampleTime=-1
  To Workspace9 : ToWorkspace  VariableName=u4  SaveFormat=Timeseries  SampleTime=-1
  wires:
  [u1] -> To Workspace6/1
  [yd] -> Mux1/1
  Mux5/1 -> Scope6/1
  [theta_d] -> Mux4/1
  [phid] -> Mux5/1
  [y] -> To Workspace1/1, Mux1/2
  [psi] -> Mux3/2, To Workspace3/1
  Mux4/1 -> Scope5/1
  [phi] -> To Workspace5/1, Mux5/2
  Mux1/1 -> Scope2/1
  [theta] -> Mux4/2, To Workspace4/1
  [psid] -> Mux3/1
  [xd] -> Mux2/1
  [zd] -> Mux/1
  Mux3/1 -> Scope4/1
  [z] -> Mux/2, To Workspace/1
  Mux2/1 -> Scope3/1
  Mux/1 -> Scope1/1
  [x] -> To Workspace2/1, Mux2/2
  [u2] -> To Workspace7/1
  [u3] -> To Workspace8/1
  [u4] -> To Workspace9/1
  [epsilonz] -> To Workspace11/1
  [w_psi] -> To Workspace10/1
  [wz] -> To Workspace12/1
  [epsilon_psi] -> To Workspace13/1

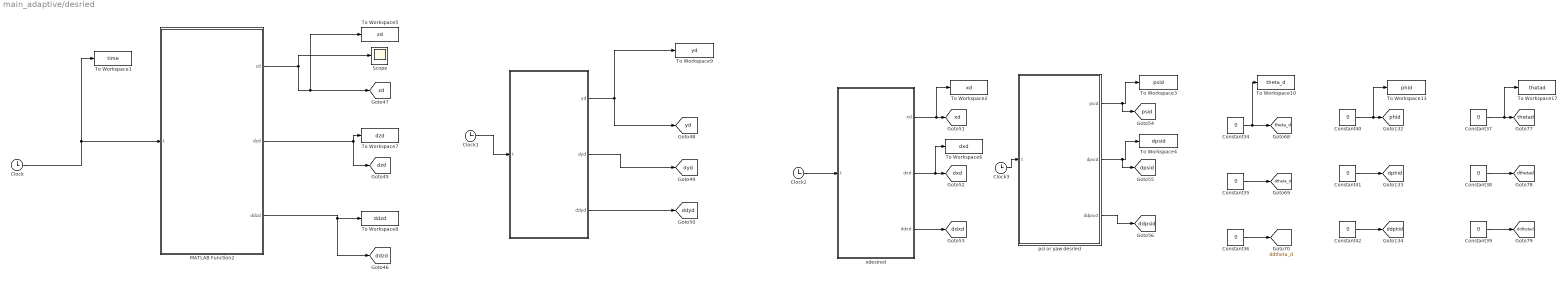
== system main_adaptive/desried ==
  " " : MATLAB Function  TreatAsAtomicUnit=on
  " xdesired" : MATLAB Function  TreatAsAtomicUnit=on
  Clock{,1..3} (4 alike) : Clock
  Constant{34..42} (9 alike) : Constant  Value=0
  MATLAB Function2 : MATLAB Function  TreatAsAtomicUnit=on
  Scope : Scope
  To Workspace1 : ToWorkspace  VariableName=time  SampleTime=-1
      settings: Save2DSignal=2-D array (concatenate along first dimension)
  To Workspace10 : ToWorkspace  VariableName=theta_d  SaveFormat=Timeseries  SampleTime=20
      settings: Save2DSignal=2-D array (concatenate along first dimension)
  To Workspace13 : ToWorkspace  VariableName=phid  SaveFormat=Timeseries  SampleTime=20
      settings: Save2DSignal=2-D array (concatenate along first dimension)
  To Workspace17 : ToWorkspace  VariableName=thetad  SampleTime=-1
      settings: Save2DSignal=2-D array (concatenate along first dimension)
  To Workspace2 : ToWorkspace  VariableName=xd  SampleTime=-1
      settings: Save2DSignal=2-D array (concatenate along first dimension)
  To Workspace3 : ToWorkspace  VariableName=psid  SampleTime=-1
      settings: Save2DSignal=2-D array (concatenate along first dimension)
  To Workspace4 : ToWorkspace  VariableName=dpsid  SampleTime=-1
      settings: Save2DSignal=2-D array (concatenate along first dimension)
  To Workspace5 : ToWorkspace  VariableName=zd  SampleTime=-1
      settings: Save2DSignal=2-D array (concatenate along first dimension)
  To Workspace6 : ToWorkspace  VariableName=dxd  SampleTime=-1
      settings: Save2DSignal=2-D array (concatenate along first dimension)
  To Workspace7 : ToWorkspace  VariableName=dzd  SampleTime=-1
      settings: Save2DSignal=2-D array (concatenate along first dimension)
  To Workspace8 : ToWorkspace  VariableName=ddzd  SampleTime=-1
      settings: Save2DSignal=2-D array (concatenate along first dimension)
  To Workspace9 : ToWorkspace  VariableName=yd  SampleTime=-1
      settings: Save2DSignal=2-D array (concatenate along first dimension)
  psi or yaw desried : MATLAB Function  TreatAsAtomicUnit=on
  tag scope: ddphid=global, ddpsid=global, ddtheta_d=global, ddthetad=global, ddxd=global, ddyd=global, ddzd=global, dphid=global, dpsid=global, dtheta_d=global, dthetad=global, dxd=global, dyd=global, dzd=global, phid=global, psid=global, theta_d=global, thetad=global, xd=global, yd=global, zd=global
  wires:
  Constant40/1 -> To Workspace13/1, [phid]
  " xdesired"/1(xd) -> To Workspace2/1, [xd]
  Constant34/1 -> To Workspace10/1, [theta_d]
  Clock2/1 -> " xdesired"/1(t)
  Constant36/1 -> [ddtheta_d]
  Constant41/1 -> [dphid]
  MATLAB Function2/2(dzd) -> [dzd], To Workspace7/1
  Constant37/1 -> To Workspace17/1, [thetad]
  Constant38/1 -> [dthetad]
  " "/3(ddyd) -> [ddyd]
  " xdesired"/3(ddxd) -> [ddxd]
  " "/2(dyd) -> [dyd]
  MATLAB Function2/1(zd) -> To Workspace5/1, [zd], Scope/1
  " "/1(yd) -> [yd], To Workspace9/1
  " xdesired"/2(dxd) -> To Workspace6/1, [dxd]
  MATLAB Function2/3(ddzd) -> [ddzd], To Workspace8/1
  psi or yaw desried/2(dpsid) -> [dpsid], To Workspace4/1
  psi or yaw desried/1(psid) -> [psid], To Workspace3/1
  Constant42/1 -> [ddphid]
  Clock/1 -> To Workspace1/1, MATLAB Function2/1(t)
  Clock3/1 -> psi or yaw desried/1(t)
  Constant35/1 -> [dtheta_d]
  Constant39/1 -> [ddthetad]
  Clock1/1 -> " "/1(t)
  psi or yaw desried/3(ddpsid) -> [ddpsid]

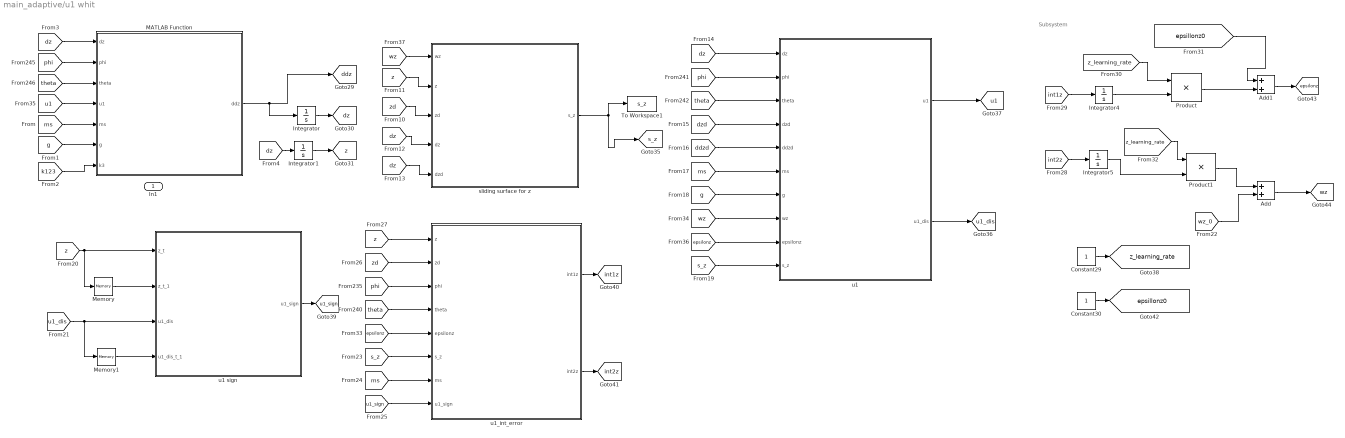
== system main_adaptive/u1 whit  ==
  note: Subsystem
  In1 : Inport
  Add : Sum
  Add1 : Sum
  Constant29 : Constant
  Constant30 : Constant
  Integrator{,1,4..5} (4 alike) : Integrator
  MATLAB Function : MATLAB Function  TreatAsAtomicUnit=on
  Memory : Memory
  Memory1 : Memory
  Product : Product
  Product1 : Product
  To Workspace1 : ToWorkspace  VariableName=s_z  SampleTime=-1
      settings: Save2DSignal=2-D array (concatenate along first dimension)
  sliding surface for z : MATLAB Function  TreatAsAtomicUnit=on
  u1 : MATLAB Function  TreatAsAtomicUnit=on
  u1 sign : MATLAB Function  TreatAsAtomicUnit=on
  u1_int_error : MATLAB Function  TreatAsAtomicUnit=on
  tag scope: ddz=global, dz=global, epsillonz0=global, epsilonz=global, int1z=global, int2z=global, s_z=global, u1=global, u1_dis=global, u1_sign=global, wz=global, z=global, z_learning_rate=global
  wires:
  [theta] -> u1/3(theta)
  [zd] -> u1_int_error/2(zd)
  [ddzd] -> u1/5(ddzd)
  [zd] -> sliding surface for z/3(zd)
  [z] -> Memory/1, u1 sign/1(z_t)
  [s_z] -> u1/10(s_z)
  [s_z] -> u1_int_error/6(s_z)
  [u1_dis] -> Memory1/1, u1 sign/3(u1_dis)
  u1 sign/1(u1_sign) -> [u1_sign]
  [wz] -> sliding surface for z/1(wz)
  [epsilonz] -> u1_int_error/5(epsilonz)
  [ms] -> u1_int_error/7(ms)
  [g] -> u1/7(g)
  [z] -> u1_int_error/1(z)
  [dz] -> sliding surface for z/4(dz)
  [dz] -> u1/1(dz)
  [z] -> sliding surface for z/2(z)
  u1/2(u1_dis) -> [u1_dis]
  u1_int_error/2(int2z) -> [int2z]
  [theta] -> u1_int_error/4(theta)
  [phi] -> u1_int_error/3(phi)
  [u1_sign] -> u1_int_error/8(u1_sign)
  Memory1/1 -> u1 sign/4(u1_dis_t_1)
  u1/1(u1) -> [u1]
  sliding surface for z/1(s_z) -> [s_z], To Workspace1/1
  Memory/1 -> u1 sign/2(z_t_1)
  u1_int_error/1(int1z) -> [int1z]
  [epsilonz] -> u1/9(epsilonz)
  [dzd] -> u1/4(dzd)
  [ms] -> u1/6(ms)
  [phi] -> u1/2(phi)
  [wz] -> u1/8(wz)
  [dz] -> sliding surface for z/5(dzd)
  Product/1 -> Add1/2
  Add/1 -> [wz]
  [int1z] -> Integrator4/1
  Integrator5/1 -> Product1/2
  [z_learning_rate] -> Product1/1
  Constant30/1 -> [epsillonz0]
  Integrator4/1 -> Product/2
  Constant29/1 -> [z_learning_rate]
  [epsillonz0] -> Add1/1
  [z_learning_rate] -> Product/1
  [int2z] -> Integrator5/1
  Product1/1 -> Add/1
  Add1/1 -> [epsilonz]
  [wz_0] -> Add/2
  Integrator1/1 -> [z]
  [k123] -> MATLAB Function/7(k3)
  [ms] -> MATLAB Function/5(ms)
  [g] -> MATLAB Function/6(g)
  [u1] -> MATLAB Function/4(u1)
  MATLAB Function/1(ddz) -> [ddz], Integrator/1
  Integrator/1 -> [dz]
  [theta] -> MATLAB Function/3(theta)
  [dz] -> MATLAB Function/1(dz)
  [dz] -> Integrator1/1
  [phi] -> MATLAB Function/2(phi)

== matlab function main_adaptive/u1 whit /u1_int_error ==
  data: z input; zd input; int1z output; phi input; theta input; epsilonz input; s_z input; ms input; u1_sign input; int2z output
function [int1z,int2z] = int_error_z(z,zd,phi,theta,epsilonz,s_z,ms,u1_sign)
%   equation 22
int1z = u1_sign*ms*(zd - z)*tanh(s_z)/(cos(theta)*cos(phi));

%   equation 22
int2z = u1_sign*(4*ms*epsilonz*(zd - z)^2*exp(-2*s_z))/(cos(theta)*cos(phi)*(1 + exp(-2*s_z))^2);
end

== matlab function main_adaptive/desried/psi or yaw desried ==
  data: t input; psid output; dpsid output; ddpsid output
function [psid,dpsid,ddpsid] = psi_desried(t)
%   equation 59
if (t <= 60)
    psid = 0.5;
else
    psid = 0;
end

dpsid = 0;
ddpsid = 0;
end

== matlab function main_adaptive/Subsystem1/sliding surface for psi ==
  data: w_psi input; s_psi output; psi input; psid input; dpsi input; dpsid input
function s_psi = sliding_sur_psi(w_psi,psi,psid,dpsi,dpsid)

s_psi=w_psi*(psid-psi)+(dpsid-dpsi);

end

== matlab function main_adaptive/Subsystem1/u4 ==
  data: dpsi input; dpsid input; u4 output; ddpsid input; c input; Iz input; eps_psi input; w_psi input; s_psi input; u4_dis output
function [u4,u4_dis] = u4_function(dpsi,dpsid,ddpsid,c,Iz,eps_psi,w_psi,s_psi)
u4_dis = Iz/c*(eps_psi*tanh(s_psi));
u4 = Iz/c*(w_psi*(dpsid - dpsi) + ddpsid) + Iz/c*(eps_psi*tanh(s_psi));
end

== matlab function main_adaptive/Subsystem1/int error u4 ==
  data: psi input; psid input; int1psi output; s_psi input; Iz input; c input; epsilon_psi input; u4_sign input; int2psi output
function [int1psi,int2psi] = int_error_psi(psi,psid,s_psi,Iz,c,epsilon_psi,u4_sign)
%   equation 22
int1psi = u4_sign*Iz*(psid - psi)*tanh(s_psi)/c;

%   equation 22
int2psi = u4_sign*(4*Iz*epsilon_psi*(psid - psi)^2*exp(-2*s_psi))/(c*(1 + exp(-2*s_psi))^2);
end

== matlab function main_adaptive/Subsystem1/u4 sign  ==
  data: psi_t input; psi_t_1 input; u4_sign output; u4_dis input; u4_dis_t_1 input
function u4_sign  = u4_sing(psi_t,psi_t_1,u4_dis,u4_dis_t_1)
if u4_dis-u4_dis_t_1==0
    u4_sign=0;
else
u4_sign=sign( (psi_t-psi_t_1)/(u4_dis-u4_dis_t_1) );
end

== matlab function main_adaptive/desried/ xdesired ==
  data: t input; xd output; dxd output; ddxd output
function [xd,dxd,ddxd] = xdesired(t)

% if (t <= 10 || t > 30)
%     xd = 0.6;
% else
%     xd = 0.3;
% end
% 
% dxd = 0;
% ddxd = 0;
% end

 xd=0.6*sin(t);
 dxd=0.6*cos(t);
 ddxd=-0.6*sin(t);

== matlab function main_adaptive/Subsystem2/theta & x ==
  data: v input; thetad input; dv output; phi input; psi input; u1 input; a1 input; a2 input; a3 input; ms input
function dv = fcn(v,thetad,phi,psi,u1,a1,a2,a3,ms)
%   equation 36
A = [0,1,0
    -a1*(cos(thetad)*cos(phi)*cos(psi))*u1/ms + a2*a3/a1,a2/a1-a3,a2^2/a1
    -a3/a1,-1/a1,-a2/a1];
dv = A*v;
end

== matlab function main_adaptive/desried/  ==
  data: t input; yd output; dyd output; ddyd output
function [yd,dyd,ddyd] = ydesired(t)
% 
% if (t <= 20 || t > 40)
%   yd = 0.6;
%     dyd = 0;
%     ddyd = 0;
% else
%     yd = 0.3;
%     dyd = 0;
%     ddyd = 0;
% end
% 
% 


  yd=0.6*cos(t);
  dyd=-0.6*sin(t);
  ddyd=-0.6*cos(t);

end

== matlab function main_adaptive/Subsystem2/MATLAB Function4 ==
  data: dx input; s_theta output; x input; dtheta input; theta input; dxd input; xd input; dtheta_d input; theta_d input; alpha1 input; alpha2 input; alpha3 input
function s_theta  = s_theta(dx,x,dtheta,theta,dxd,xd,dtheta_d,theta_d,alpha1,alpha2,alpha3)
%   equation 30
s_theta = alpha1*(dxd-dx) + alpha2*(xd-x) + (dtheta_d-dtheta) + alpha3*(theta_d-theta);

== matlab function main_adaptive/Subsystem2/MATLAB Function5 ==
  data: dtheta input; theta input; dtheta_d input; ddtheta_d input; dx input; u3 output; dxd input; ddxd input; phi input; psi input; ms input; l input; Iy input; epstheta input; alpha1 input; alpha2 input; alpha3 input; s_theta input; u1 input; u3_dis output
function [u3,u3_dis] = u3_function(dtheta,theta,dtheta_d,ddtheta_d,dx,dxd,ddxd,phi,psi,ms,l,Iy,epstheta,alpha1,alpha2,alpha3,s_theta,u1)

u3_dis = Iy/l*(epstheta*tanh(s_theta));
u3 = Iy/l*(alpha1*(ddxd-((sin(theta)*cos(phi)*cos(psi)+sin(phi)*sin(psi))/ms*u1))+alpha2*(dxd-dx)+ddtheta_d+alpha3*(dtheta_d-dtheta));
end

== matlab function main_adaptive/Subsystem2/u3 sign 1 ==
  data: x_t input; x_t_1 input; u3_sign output; u3_dis input; u3_dis_t_1 input
function u3_sign  = u3_sing(x_t,x_t_1,u3_dis,u3_dis_t_1)
if u3_dis-u3_dis_t_1==0
    u3_sign=0;
else
u3_sign=sign( (x_t-x_t_1)/(u3_dis-u3_dis_t_1) );
end

== matlab function main_adaptive/Subsystem2/control parameters ==
  data: theta input; theta_d input; dx input; x input; dxd input; xd input; phi input; psi input; u1 input; s_theta input; ms input; Iy input; l input; epstheta input; int1_u3_epstheta output; int2_u3_w1 output; u3_sing input; int3_u3_w2 output; int4_u3_w3 output
function [int1_u3_epstheta,int2_u3_w1,int3_u3_w2,int4_u3_w3] = fcn(theta,theta_d,dx,x,dxd,xd,phi,psi,u1,s_theta,ms,Iy,l,epstheta,u3_sing)
%   equation 45
int1_u3_epstheta = u3_sing*(Iy*(xd-x)*tanh(s_theta))/l;

%   equation 46
int2_u3_w1 = u3_sing*(4*Iy*ms*epstheta*(xd-x)*(dxd-dx)*exp(-2*s_theta))/(l*cos(theta_d)*cos(phi)*cos(psi)*(1+exp(-2*s_theta))^2*u1+eps);

%   equation 47
int3_u3_w2 = u3_sing*(4*Iy*ms*epstheta*(xd-x)^2*exp(-2*s_theta))/(l*cos(theta_d)*cos(phi)*cos(psi)*(1+exp(-2*s_theta))^2*u1+eps);

%   equation 48
int4_u3_w3 = u3_sing*(4*Iy*epstheta*(xd-x)*(theta_d-theta)*exp(-2*s_theta))/(l*(1+exp(-2*s_theta))^2+eps);
end

== matlab function main_adaptive/Subsystem2/a1,a2,a3 ==
  data: theta_d input; phi input; alpha1 output; psi input; u1 input; w1 input; w2 input; w3 input; alpha2 output; alpha3 output; ms input
function [alpha1,alpha2,alpha3] = alpha_cal(theta_d,phi,psi,u1,w1,w2,w3,ms)
alpha1 = w1*ms/((cos(theta_d)*cos(phi)*cos(psi))*u1);
alpha2 = w2*ms/((cos(theta_d)*cos(phi)*cos(psi))*u1);
alpha3 = w3;
end

== matlab function main_adaptive/Subsystem3/phi & y ==
  data: v input; theta input; dv output; phid input; psi input; u1 input; a4 input; a5 input; a6 input; ms input
function dv = fcn(v,theta,phid,psi,u1,a4,a5,a6,ms)
%   equation 36
A = [0,1,0
    a4*(sin(phid)*sin(theta)*sin(psi)+cos(phid)*cos(psi))*u1/ms+a5*a6/a4,a5/a4-a6,a5^2/a4
    -a6/a4,-1/a4,-a5/a4];
dv = A*v;
end

== matlab function main_adaptive/Subsystem3/MATLAB Function7 ==
  data: dy input; s_phi output; y input; dphi input; phi input; dyd input; yd input; dphid input; phid input; a4 input; a5 input; a6 input
function s_phi  = s_phi(dy,y,dphi,phi,dyd,yd,dphid,phid,a4,a5,a6)
%   equation 50
s_phi = a4*(dyd-dy) + a5*(yd-y) + (dphid-dphi) + a6*(phid-phi);
end

== matlab function main_adaptive/Subsystem3/MATLAB Function8 ==
  data: dphi input; phi input; dphid input; ddphid input; dy input; dyd input; ddyd input; theta input; u2 output; psi input; ms input; l input; Ix input; epsphi input; a4 input; a5 input; a6 input; sphi input; u1 input; u2_dis output
function [u2,u2_dis] = fcn(dphi,phi,dphid,ddphid,dy,dyd,ddyd,theta,psi,ms,l,Ix,epsphi,a4,a5,a6,sphi,u1)
%   equation 14
u2_dis = Ix/l*(epsphi*tanh(sphi));
u2 = Ix/l*(a4*(ddyd-((sin(theta)*cos(phi)*sin(psi)-sin(phi)*cos(psi))/ms*u1))+a5*(dyd-dy)+ddphid+a6*(dphid-dphi));
end

== matlab function main_adaptive/Subsystem3/a4,a5,a6 ==
  data: phid input; theta input; alpha4 output; psi input; u1 input; w4 input; w5 input; w6 input; alpha5 output; alpha6 output; ms input
function [alpha4,alpha5,alpha6] = alpha_cal(phid,theta,psi,u1,w4,w5,w6,ms)
alpha4 = -w4*ms/((sin(theta)*sin(phid)*sin(psi)+cos(phid)*cos(psi))*u1);
alpha5 = -w5*ms/((sin(theta)*sin(phid)*sin(psi)+cos(phid)*cos(psi))*u1);
alpha6 = w6;
end

== matlab function main_adaptive/desried/MATLAB Function2 ==
  data: zd output; t input; dzd output; ddzd output
function [zd,dzd,ddzd]  = zdesired(t)

% if (t <= 80)
% %     zd = 0.6;
% %     dzd = 0;
% %     ddzd = 0;
   zd=0.6+0.5*sin(t);
   dzd = 0.5*cos(t);
   ddzd = -0.5*sin(t);
% else
%     zd = 0;
%     dzd = 0;
%     ddzd = 0;
% end
% 

end

== matlab function main_adaptive/Subsystem3/control parameters1 ==
  data: phi input; phid input; dy input; y input; dyd input; yd input; theta input; psi input; u1 input; sphi input; ms input; Ix input; l input; epsphi input; int1 output; int2 output; sign_y_u2dis input; int3 output; int4 output
function [int1,int2,int3,int4] = fcn(phi,phid,dy,y,dyd,yd,theta,psi,u1,sphi,ms,Ix,l,epsphi,sign_y_u2dis)
%   equation 45
int1 = sign_y_u2dis*(Ix*(yd-y)*tanh(sphi))/l;

%   equation 46
int2 = sign_y_u2dis*(4*Ix*ms*epsphi*(yd-y)*(dyd-dy)*exp(-2*sphi))/(l*(sin(theta)*sin(phid)*sin(psi)+cos(phid)*cos(psi))*(1+exp(-2*sphi))^2*u1+eps);

%   equation 47
int3 = sign_y_u2dis*(4*Ix*ms*epsphi*(yd-y)^2*exp(-2*sphi))/(l*(sin(theta)*sin(phid)*sin(psi)+cos(phid)*cos(psi))*(1+exp(-2*sphi))^2*u1+eps);

%   equation 48
int4 = sign_y_u2dis*(4*Ix*epsphi*(yd-y)*(phid-phi)*exp(-2*sphi))/(l*(1+exp(-2*sphi))^2+eps);
end
